simulink model "PI2GDL_Z"  (R2018a)
settings: Solver=VariableStepAuto  StartTime=0.0  StopTime=200.0  RelTol=1e-3
values from neighbouring files (symbols this model uses):
  B = (T*tc)/(Ti)    (= 0.482939903103)    [Controlador2GDL.m]    (also in Examen2.m)
  k = 9.22    [Controlador2GDL.m]    (also in ControladorAlfaroPI1GDL_ControlEstricto.m; ControladorAlfaroPI1GDL_ControlSuave.m; Examen2.m)
  Kp = (a)/(k*(tc+to).^2)    [Controlador2GDL.m]    (also in ControladorAlfaroPI1GDL_ControlEstricto.m = 0.669122125129; ControladorAlfaroPI1GDL_ControlSuave.m = 0.469559386056; Examen2.m)
  L = 3.17    [Controlador2GDL.m]    (also in ControladorAlfaroPI1GDL_ControlEstricto.m; ControladorAlfaroPI1GDL_ControlSuave.m; Examen2.m)
  T = 34.31    [Controlador2GDL.m]    (also in ControladorAlfaroPI1GDL_ControlEstricto.m; ControladorAlfaroPI1GDL_ControlSuave.m; Examen2.m)
  Ti = T*(a/(1+to))    (= 14.2088072572)    [Controlador2GDL.m]    (also in ControladorAlfaroPI1GDL_ControlEstricto.m = 0.0291460215681; ControladorAlfaroPI1GDL_ControlSuave.m = 0.0291460215681; Examen2.m)
  Ts = 0.1    [Examen2.m]
settings Model: Creator=wivill  LastModifiedBy=wivill

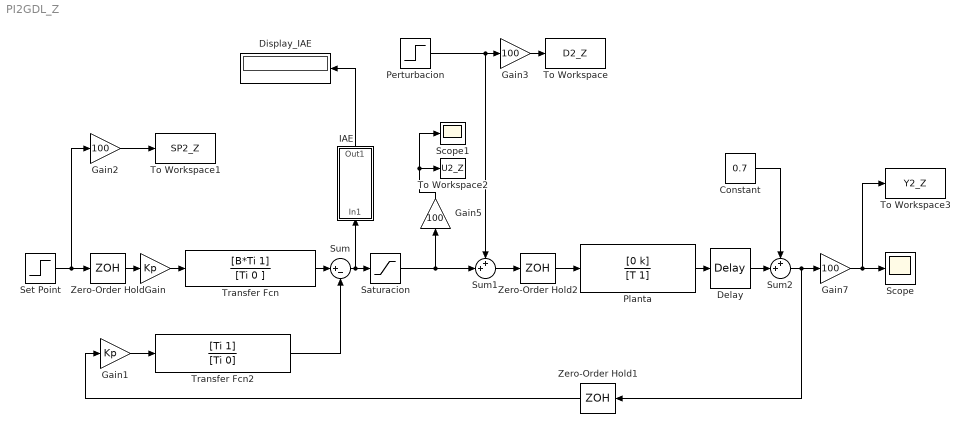
== system PI2GDL_Z ==
  Constant : Constant  Value=0.7
  Delay : TransportDelay  DelayTime=L
  "Display_IAE " : Display
  Gain : Gain  Gain=Kp
  Gain1 : Gain  Gain=Kp
  Gain{2..3,5,7} (4 alike) : Gain  Gain=100
  IAE : Subsystem
      mask help:
      | IAE performacne index
      |
      | output = int |input| dt
      mask Display:
      | disp('IAE')
      | port_label('input',1,'e')
      | port_label('output',1,'iae')
  Perturbacion : Step  Time=75  After=-0.05  SampleTime=Ts
  Planta : TransferFcn  Numerator=[0 k]  Denominator=[T 1]
  "Saturacion " : Saturate  UpperLimit=1  LowerLimit=-0.1
  Scope : Scope
  Scope1 : Scope
  "Set Point " : Step  Time=0  Before=0.7  After=0.8  SampleTime=Ts
  Sum : Sum  Inputs=|+-
  Sum1 : Sum  Inputs=++|
  Sum2 : Sum  Inputs=++|
  To Workspace : ToWorkspace  VariableName=D2_Z  SaveFormat=Timeseries  SampleTime=Ts
  To Workspace1 : ToWorkspace  VariableName=SP2_Z  SaveFormat=Timeseries  SampleTime=Ts
  To Workspace2 : ToWorkspace  VariableName=U2_Z  SaveFormat=Timeseries  SampleTime=Ts
  To Workspace3 : ToWorkspace  VariableName=Y2_Z  SaveFormat=Timeseries  SampleTime=Ts
  Transfer Fcn : TransferFcn  Numerator=[B*Ti 1]  Denominator=[Ti 0 ]
  Transfer Fcn2 : TransferFcn  Numerator=[Ti 1]  Denominator=[Ti 0]
  Zero-Order Hold : ZeroOrderHold  SampleTime=Ts
  Zero-Order Hold1 : ZeroOrderHold  SampleTime=Ts
  Zero-Order Hold2 : ZeroOrderHold  SampleTime=Ts
  wires:
  Gain2/1 -> To Workspace1/1
  "Set Point "/1 -> Zero-Order Hold/1, Gain2/1
  Gain3/1 -> To Workspace/1
  IAE/1(Out1) -> "Display_IAE "/1
  Gain1/1 -> Transfer Fcn2/1
  Transfer Fcn2/1 -> Sum/2
  "Saturacion "/1 -> Gain5/1, Sum1/2
  Perturbacion/1 -> Sum1/1, Gain3/1
  Transfer Fcn/1 -> Sum/1
  Gain/1 -> Transfer Fcn/1
  Gain7/1 -> Scope/1, To Workspace3/1
  Sum/1 -> "Saturacion "/1, IAE/1(In1)
  Sum1/1 -> Zero-Order Hold2/1
  Planta/1 -> Delay/1
  Delay/1 -> Sum2/2
  Sum2/1 -> Gain7/1, Zero-Order Hold1/1
  Constant/1 -> Sum2/1
  Zero-Order Hold/1 -> Gain/1
  Zero-Order Hold1/1 -> Gain1/1
  Zero-Order Hold2/1 -> Planta/1
  Gain5/1 -> To Workspace2/1, Scope1/1

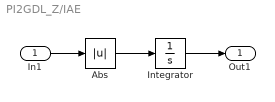
== system PI2GDL_Z/IAE ==
  In1 : Inport
  Abs : Abs
  Integrator : Integrator
  Out1 : Outport
  wires:
  In1/1 -> Abs/1
  Integrator/1 -> Out1/1
  Abs/1 -> Integrator/1
